simulink model "model2_2020"  (R2020a)
settings: Solver=VariableStepAuto  StartTime=0.0  StopTime=10.0  RelTol=1e-3
values from neighbouring files (symbols this model uses):
  A = [0, 1; -7, -5]    [domaci2.m]
  B = [0; 2]    [domaci2.m]
  K = acker(A, B, [-3, -3])    [domaci2.m]
  kr = 1 / (dcgain(s * G0 / s))    [domaci2.m]
  x0 = [-2; 2]    [domaci2.m]
settings Model: Creator=Nenad  LastModifiedBy=Nenad

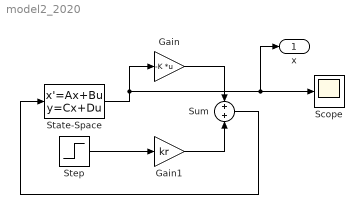
== system model2_2020 ==
  Gain : Gain  Gain=-K  Multiplication=Matrix(K*u) (u vector)
  Gain1 : Gain  Gain=kr
  Scope : Scope
  State-Space : StateSpace  A=A  B=B  C=[1, 0; 0, 1]  D=[0; 0]  InitialCondition=x0
  Step : Step  Time=0  After=5  SampleTime=0
  Sum : Sum  Inputs=+|+
  x : Outport  SignalName=x
  wires:
  State-Space/1 -> x/1, Scope/1, Gain/1
  Step/1 -> Gain1/1
  Gain/1 -> Sum/1
  Gain1/1 -> Sum/2
  Sum/1 -> State-Space/1
